simulink model "crazyflie"  (R2018b)
settings: Solver=FixedStepDiscrete  StartTime=0.0  StopTime=10  FixedStep=0.01  RelTol=1e-3
values from neighbouring files (symbols this model uses):
  FF_pitch = zeros(:,2)    [linear_manual.m]
  g = 9.81    [linear_manual.m]
  Kang = K(:, [1 2 3 4])    [linear_manual.m]
  Kr_pitch = K(:,end)    [linear_manual.m]
  Ts = 0.01    [linear_manual.m]
undefined symbols (not defined in the file or in its folder): DiscIntNeverNeededParam
settings Model: PauseTimes=7  Creator=Zrean  LastModifiedBy=Johan
settings OptimizationCC: DefaultParameterBehavior=Inlined  UseDivisionForNetSlopeComputation=on  UseFloatMulNetSlope=on  UseSpecifiedMinMax=on  InlineInvariantSignals=on  PassReuseOutputArgsAs=Individual arguments  ZeroExternalMemoryAtStartup=off  ZeroInternalMemoryAtStartup=off  NoFixptDivByZeroProtection=on  EfficientFloat2IntCast=on  LifeSpan=1
settings DebuggingCC: AlgebraicLoopMsg=error  ParameterTunabilityLossMsg=error
settings HardwareCC: ProdBitPerPointer=32  ProdBitPerSizeT=32  ProdBitPerPtrDiffT=32  ProdLargestAtomicInteger=Long  ProdLargestAtomicFloat=Double  ProdWordSize=32  ProdHWDeviceType=ARM Compatible->ARM Cortex
settings SFSimCC: SimUseLocalCustomCode=off  MATLABDynamicMemAlloc=off
settings RTWCC: SystemTargetFile=ert.tlc  GenCodeOnly=on  TemplateMakefile=ert_default_tmf  GenerateReport=on  RTWUseLocalCustomCode=off  BuildConfiguration=Faster Runs  IncludeHyperlinkInReport=on  LaunchReport=on  GenerateTraceInfo=on  GenerateTraceReport=on  GenerateTraceReportSl=on  GenerateTraceReportSf=on  GenerateTraceReportEml=on  GenerateCodeMetricsReport=on
settings CodeAppCC: ForceParamTrailComments=on  IgnoreCustomStorageClasses=off  OperatorAnnotations=on  SimulinkDataObjDesc=on  SFDataObjDesc=on  MATLABFcnDesc=on  CustomSymbolStrGlobalVar=rt$N$M  CustomSymbolStrType=$N$M  CustomSymbolStrFcn=$N$M$F  CustomSymbolStrMacro=$N$M  InsertBlockDesc=on  StateflowObjectComments=on  MATLABSourceComments=on
settings ERTTargetCC: TargetLangStandard=C99 (ISO)  MultiwordLength=2048  CombineSignalStateStructs=on  SuppressErrorStatus=on  SupportAbsoluteTime=off  SupportNonFinite=off  SupportComplex=off  InlinedParameterPlacement=NonHierarchical  ERTCustomFileTemplate=crazyflie_wrapper.tlc  ERTFilePackagingFormat=CompactWithDataFile
settings SimscapeCC: SimscapeNormalizeSystem=off

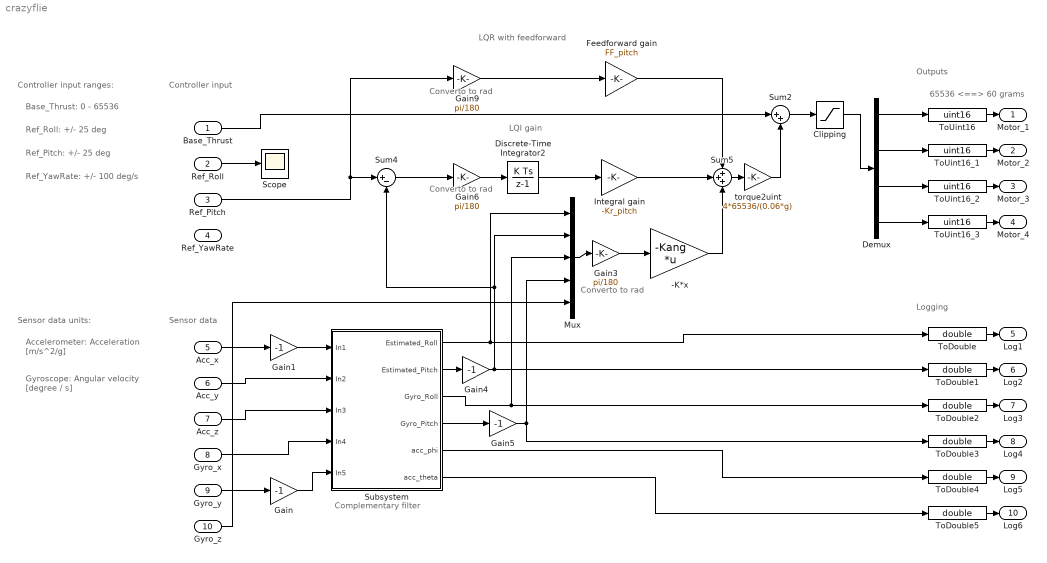
== system crazyflie ==
  note: Complementary filter
  note: Converto to rad
  note: Converto to rad
  note: Converto to rad
  note: LQI gain
  note: LQR with feedforward
  note: 65536 <==> 60 grams
  note: Logging
  note: Outputs
  note: Sensor data
  note: Controller input
  note: Ref_Roll: +/- 25 deg
  note: Base_Thrust: 0 - 65536
  note: Ref_Pitch: +/- 25 deg
  note: Ref_YawRate: +/- 100 deg/s
  note: Controller input ranges:
  note: Gyroscope:
      | Angular velocity [degree / s]
  note: Accelerometer:
      | Acceleration [m/s^2/g]
  note: Sensor data units:
  Base_Thrust : Inport
  Ref_Roll : Inport  Port=2  OutDataTypeStr=double
  Ref_Pitch : Inport  Port=3
  Ref_YawRate : Inport  Port=4  OutDataTypeStr=double
  Acc_x : Inport  Port=5  OutDataTypeStr=double  PortDimensions=1
  Acc_y : Inport  Port=6  OutDataTypeStr=double  PortDimensions=1
  Acc_z : Inport  Port=7  OutDataTypeStr=double  PortDimensions=1
  Gyro_x : Inport  Port=8  OutDataTypeStr=double  PortDimensions=1
  Gyro_y : Inport  Port=9  OutDataTypeStr=double  PortDimensions=1
  Gyro_z : Inport  Port=10  OutDataTypeStr=double  PortDimensions=1
  -K*x : Gain  Gain=-Kang  Multiplication=Matrix(K*u) (u vector)
  Clipping : Saturate  UpperLimit=65000  LowerLimit=0
  Demux : Demux
  Discrete-Time Integrator2 : DiscreteIntegrator  SampleTime=Ts  ICPrevOutput=DiscIntNeverNeededParam  ICPrevScaledInput=DiscIntNeverNeededParam
  Feedforward gain : Gain  Gain=FF_pitch
  Gain{,1,4..5} (4 alike) : Gain  Gain=-1
  Gain3 : Gain  Gain=pi/180
  Gain6 : Gain  Gain=pi/180
  Gain9 : Gain  Gain=pi/180
  Integral gain : Gain  Gain=-Kr_pitch
  Mux : Mux  Inputs=5
  Scope : Scope
  Subsystem : Subsystem
  Sum2 : Sum  Inputs=|++
  Sum4 : Sum  Inputs=|+-
  Sum5 : Sum  Inputs=+++
  ToDouble{,1..5} (6 alike) : DataTypeConversion  OutDataTypeStr=double  SaturateOnIntegerOverflow=on
  ToUint16 : DataTypeConversion  OutDataTypeStr=uint16  SaturateOnIntegerOverflow=on
  ToUint16_1 : DataTypeConversion  OutDataTypeStr=uint16  SaturateOnIntegerOverflow=on
  ToUint16_2 : DataTypeConversion  OutDataTypeStr=uint16  SaturateOnIntegerOverflow=on
  ToUint16_3 : DataTypeConversion  OutDataTypeStr=uint16  SaturateOnIntegerOverflow=on
  torque2uint : Gain  Gain=4*65536/(0.06*g)
  Motor_1 : Outport  OutDataTypeStr=uint16  LockScale=on
  Motor_2 : Outport  Port=2  OutDataTypeStr=uint16  LockScale=on
  Motor_3 : Outport  Port=3  OutDataTypeStr=uint16  LockScale=on
  Motor_4 : Outport  Port=4  OutDataTypeStr=uint16  LockScale=on
  Log1 : Outport  Port=5  OutDataTypeStr=double
  Log2 : Outport  Port=6  OutDataTypeStr=double
  Log3 : Outport  Port=7  OutDataTypeStr=double
  Log4 : Outport  Port=8  OutDataTypeStr=double
  Log5 : Outport  Port=9  OutDataTypeStr=double
  Log6 : Outport  Port=10  OutDataTypeStr=double
  wires:
  ToUint16/1 -> Motor_1/1
  ToUint16_1/1 -> Motor_2/1
  ToUint16_2/1 -> Motor_3/1
  ToUint16_3/1 -> Motor_4/1
  ToDouble/1 -> Log1/1
  ToDouble1/1 -> Log2/1
  ToDouble2/1 -> Log3/1
  ToDouble3/1 -> Log4/1
  ToDouble4/1 -> Log5/1
  ToDouble5/1 -> Log6/1
  Gyro_x/1 -> Subsystem/4(In4)
  Gyro_y/1 -> Gain/1
  Demux/3 -> ToUint16_2/1
  Demux/4 -> ToUint16_3/1
  Sum5/1 -> torque2uint/1
  Demux/2 -> ToUint16_1/1
  Demux/1 -> ToUint16/1
  Subsystem/1(Estimated_Roll) -> Mux/1, ToDouble/1
  Gain4/1 -> ToDouble1/1, Sum4/2, Mux/2
  Gain5/1 -> ToDouble3/1, Mux/4
  Gain/1 -> Subsystem/5(In5)
  Acc_x/1 -> Gain1/1
  Gain3/1 -> -K*x/1
  Gain1/1 -> Subsystem/1(In1)
  Acc_y/1 -> Subsystem/2(In2)
  Acc_z/1 -> Subsystem/3(In3)
  Subsystem/4(Gyro_Pitch) -> Gain5/1
  Subsystem/2(Estimated_Pitch) -> Gain4/1
  torque2uint/1 -> Sum2/2
  Gain6/1 -> Discrete-Time Integrator2/1
  Discrete-Time Integrator2/1 -> Integral gain/1
  Sum4/1 -> Gain6/1
  Subsystem/3(Gyro_Roll) -> Mux/3, ToDouble2/1
  Mux/1 -> Gain3/1
  Sum2/1 -> Clipping/1
  Clipping/1 -> Demux/1
  Gain9/1 -> Feedforward gain/1
  Subsystem/5(acc_phi) -> ToDouble4/1
  Subsystem/6(acc_theta) -> ToDouble5/1
  Base_Thrust/1 -> Sum2/1
  Feedforward gain/1 -> Sum5/1
  Integral gain/1 -> Sum5/2
  -K*x/1 -> Sum5/3
  Ref_Roll/1 -> Scope/1
  Gyro_z/1 -> Mux/5
  Ref_Pitch/1 -> Sum4/1, Gain9/1

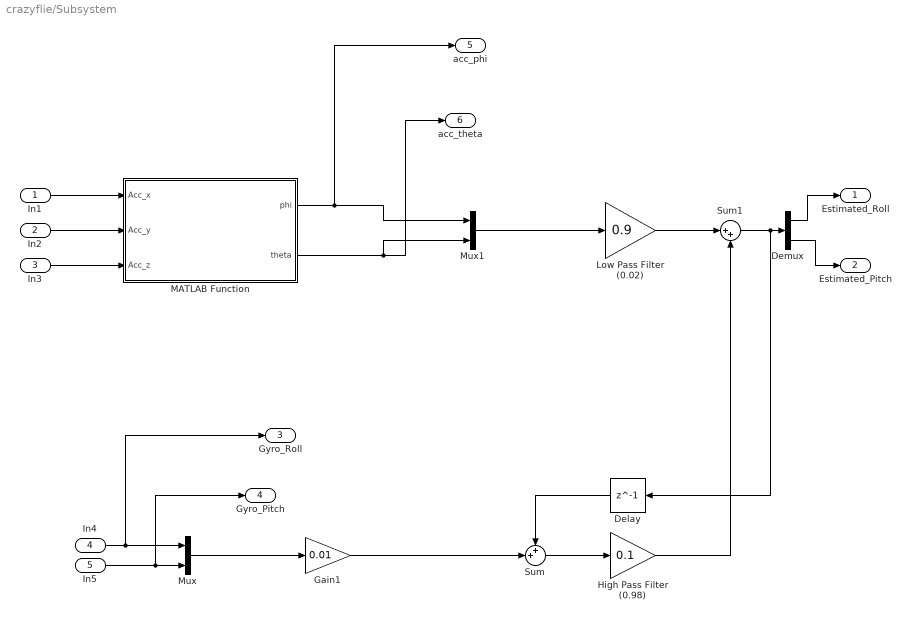
== system crazyflie/Subsystem ==
  In1 : Inport
  In2 : Inport  Port=2
  In3 : Inport  Port=3
  In4 : Inport  Port=4
  In5 : Inport  Port=5
  Delay : Delay  DelayLength=1  InitialCondition=0
  Demux : Demux  Outputs=2
  Gain1 : Gain  Gain=0.01
  High Pass Filter (0.98) : Gain  Gain=0.1
  Low Pass Filter (0.02) : Gain  Gain=0.9
  MATLAB Function : MATLAB Function  TreatAsAtomicUnit=on
  Mux : Mux  Inputs=2
  Mux1 : Mux  Inputs=2
  Sum : Sum  Inputs=++|
  Sum1 : Sum  Inputs=|++
  Estimated_Roll : Outport
  Estimated_Pitch : Outport  Port=2
  Gyro_Roll : Outport  Port=3
  Gyro_Pitch : Outport  Port=4
  acc_phi : Outport  Port=5
  acc_theta : Outport  Port=6
  wires:
  In2/1 -> MATLAB Function/2(Acc_y)
  MATLAB Function/1(phi) -> acc_phi/1, Mux1/1
  MATLAB Function/2(theta) -> acc_theta/1, Mux1/2
  Mux1/1 -> Low Pass Filter (0.02)/1
  Demux/1 -> Estimated_Roll/1
  In5/1 -> Gyro_Pitch/1, Mux/2
  Gain1/1 -> Sum/2
  Delay/1 -> Sum/1
  Sum1/1 -> Delay/1, Demux/1
  Mux/1 -> Gain1/1
  Low Pass Filter (0.02)/1 -> Sum1/1
  Sum/1 -> High Pass Filter (0.98)/1
  In4/1 -> Gyro_Roll/1, Mux/1
  In1/1 -> MATLAB Function/1(Acc_x)
  Demux/2 -> Estimated_Pitch/1
  In3/1 -> MATLAB Function/3(Acc_z)
  High Pass Filter (0.98)/1 -> Sum1/2

== matlab function crazyflie/Subsystem/MATLAB Function ==
  data: phi output; Acc_x input; theta output; Acc_y input; Acc_z input
function [phi,theta] = fcn(Acc_x,Acc_y,Acc_z)

%Normalization Part
Acceleration_Vector = [Acc_x,Acc_y,Acc_z]';
Normalized_Acceleration = Acceleration_Vector / norm(Acceleration_Vector);
fx_bar=Normalized_Acceleration(1);
fy_bar=Normalized_Acceleration(2);
fz_bar=Normalized_Acceleration(3);
%Pitch and Roll Angles
phi = atan2d(fy_bar,fz_bar);
theta = atan2d(-fx_bar,((fy_bar^2+fz_bar^2)^0.5));
end
